simulink model "Ejemplo02"  (R2021b)
settings: Solver=VariableStepAuto  StartTime=0.0  StopTime=10.0  RelTol=1e-3
settings Model: Creator=juandiegocastropadilla  LastModifiedBy=juandiegocastropadilla

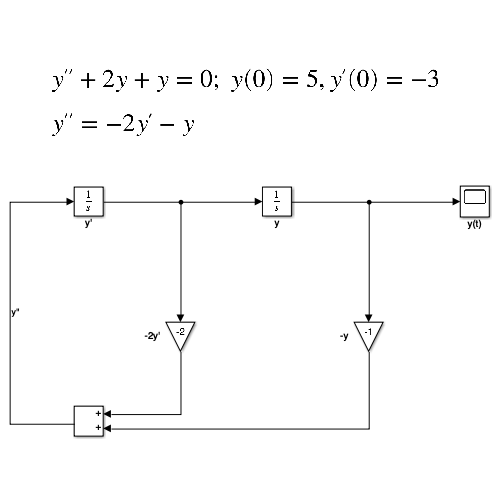
[thumbnail: Simulink's stored preview of the top-level diagram]
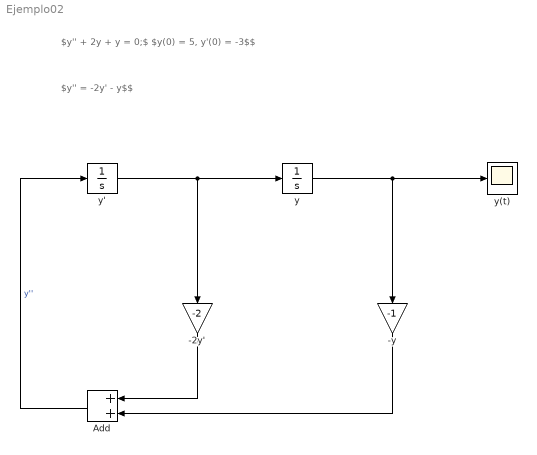
== system Ejemplo02 ==
  note: $y'' = -2y' - y$$
  note: $y'' + 2y + y = 0;$ $y(0) = 5, y'(0) = -3$$
  -2y' : Gain  Gain=-2
  -y : Gain  Gain=-1
  Add : Sum
  y : Integrator  InitialCondition=5
  y' : Integrator  InitialCondition=-3
  y(t) : Scope
  wires:
  y'/1 -> y/1, -2y'/1
  y/1 -> y(t)/1, -y/1
  -2y'/1 -> Add/1
  -y/1 -> Add/2
  Add/1 -> y'/1  "y''"
